simulink library "FunWithArduinoLib"  (R2014b)
settings: Solver=ode45  StartTime=0.0  StopTime=10.0  RelTol=1e-3
libraries: FunWithArduinoLib x1
settings Model: Creator=cgupta  LastModifiedBy=rpurser

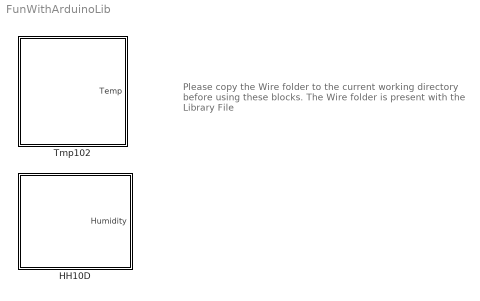
== system FunWithArduinoLib ==
  note: Please copy the Wire folder to the
      | current working directory before using
      | these blocks.
      |
      | The Wire folder is present with the Library File
  HH10D : Subsystem  mask(HH10D){interruptNum=1, sampleTime=1.2}
      mask prompts: interruptNum "Interrupt Number"; sampleTime "Sample Time"
      mask help:
      | This is the driver block for the sensor HH10D.
      | http://www.sparkfun.com/datasheets/Sensors/Temperature/HH10D.pdf
      |
      | The Interrupt Number is the interrupt you want to use on your Arduino.
      | (Arduino Uno has interrupts 0 & 1) 0 - pin D2 and 1 on pin D3
      |
      | Sample Time is the time at which you want to pull data from the Sensor.
      | This sensor needs a sample time of atleast 1 second to give meaningful data.
      mask Display: image('hh10d.jpg')
  Tmp102 : Subsystem  mask(TMP 102){deviceAddress=72, sampleTime=0.1}
      mask prompts: deviceAddress "Device Address"; sampleTime "Sample Time"
      mask help:
      | This is the driver block for Temperature Sensor TMP 102
      | http://www.sparkfun.com/datasheets/Sensors/Temperature/tmp102.pdf
      |
      | The Device Address is the i2C Address of the Temperature sensor that is by
      | default at 72.
      | You can also set the sample Time in seconds
      mask Display: image('Tmp102.jpg')

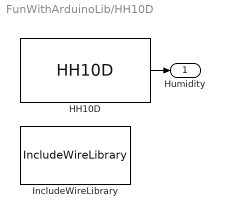
== system FunWithArduinoLib/HH10D ==
  HH10D : S-Function  InitFcn=try, set_param(gcb,'FunctionName','HH10D'), end  FunctionName=HH10D  Parameters=int8(1),1.2  SFunctionModules=HH10D_wrapper  EnableBusSupport=off  mask(S-Function Builder){}
      mask help: Simulink:masks:SFunctionBuilder_MD
      mask init:
      | val = [[.9  0.75 0.75 1 1 .9 .9 1]',[1 1 0.75 0.75 .9 .9 1 .9]'];try , sys = get_param(gcb,'SfunBuilderFcnName');if isempty(sys), sys = get_param(gcb,'FunctionName'); end,catch, sys = get_param(gcb,'FunctionName'); end
      settings: PreSaveFcn=try, set_param(gcb,'FunctionName','HH10D'), end  OpenFcn=sfunctionwizard(gcbh)
      mask Display: plot(val(:,1),val(:,2)),disp(sys), port_label('output',1,'Humidity')
  IncludeWireLibrary : FunWithArduinoLib/Tmp102/IncludeWireLibrary
  Humidity : Outport
  wires:
  HH10D/1 -> Humidity/1

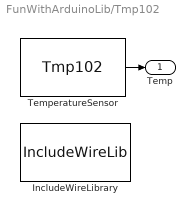
== system FunWithArduinoLib/Tmp102 ==
  IncludeWireLibrary : S-Function  InitFcn=try, set_param(gcb,'FunctionName','IncludeWireLib'), end  FunctionName=IncludeWireLib  SFunctionModules=IncludeWireLib_wrapper  EnableBusSupport=off  mask(S-Function Builder){}
      mask help: Simulink:masks:SFunctionBuilder_MD
      mask init: same as FunWithArduinoLib/HH10D/HH10D
      settings: PreSaveFcn=try, set_param(gcb,'FunctionName','IncludeWireLib'), end  OpenFcn=sfunctionwizard(gcbh)
      mask Display:
      | plot(val(:,1),val(:,2))
      | disp(sys)
  TemperatureSensor : S-Function  InitFcn=try, set_param(gcb,'FunctionName','Tmp102'), end  FunctionName=Tmp102  Parameters=int8(72),0.1  SFunctionModules=Tmp102_wrapper  EnableBusSupport=off  mask(S-Function Builder){}
      mask help: Simulink:masks:SFunctionBuilder_MD
      mask init: same as FunWithArduinoLib/HH10D/HH10D
      settings: PreSaveFcn=try, set_param(gcb,'FunctionName','Tmp102'), end  OpenFcn=sfunctionwizard(gcbh)
      mask Display: plot(val(:,1),val(:,2)),disp(sys), port_label('output',1,'Temp')
  Temp : Outport
  wires:
  TemperatureSensor/1 -> Temp/1
